simulink model "QuadrotorVertPlane_R2017b"  (R2020a)
settings: Solver=ode23s  StartTime=0.0  StopTime=20  RelTol=1e-3  EnableMultiTasking=on
values from neighbouring files (symbols this model uses):
  Acx = 4    [quadrotorparam.m]
  Acy = 4    [quadrotorparam.m]
  bt = 1    [quadrotorparam.m]
  ciLtheta = 0    [quadrotorparam.m]
  cipx = 0    [quadrotorparam.m]
  cipy = 0    [quadrotorparam.m]
  citheta = 0    [quadrotorparam.m]
  cix = 0    [quadrotorparam.m]
  ciy = 0    [quadrotorparam.m]
  g = 9.8    [quadrotorparam.m]
  J = 0.0112    [quadrotorparam.m]
  kt = 5    [quadrotorparam.m]
  kvt = 5    [quadrotorparam.m]
  kvx = .1    (= 0.1)    [quadrotorparam.m]
  kvy = 1    [quadrotorparam.m]
  kx = .5    (= 0.5)    [quadrotorparam.m]
  ky = .5    (= 0.5)    [quadrotorparam.m]
  l = 0.2    [quadrotorparam.m]
  lf = 0.2    [quadrotorparam.m]
  lr = 0.2    [quadrotorparam.m]
  m = 1    [quadrotorparam.m]
  SteptOff = 80    [quadrotorparam.m]
  SteptTc = 20    [quadrotorparam.m]
  Tcx = 30    [quadrotorparam.m]
  Tcy = 30    [quadrotorparam.m]
  txref = 1    [quadrotorparam.m]
  tyref = 1    [quadrotorparam.m]
  xref = 10    [quadrotorparam.m]
  yref = 10    [quadrotorparam.m]
settings Model: Creator=tristan  LastModifiedBy=cal
settings DataIOCC: SaveFormat=Array  SignalLoggingSaveFormat=ModelDataLogs  ReturnWorkspaceOutputs=off  OutputOption=SpecifiedOutputTimes  OutputTimes=[tStart:outputsample:tFinal]
settings OptimizationCC: ExpressionDepthLimit=2147483647  LifeSpan=inf
settings DebuggingCC: UnderspecifiedInitializationDetection=Classic  MergeDetectMultiDrivingBlocksExec=none  FcnCallInpInsideContextMsg=warning  StateNameClashWarn=warning  SFUnexpectedBacktrackingDiag=warning  SFNoUnconditionalDefaultTransitionDiag=warning  SFExecutionAtInitializationDiag=none  ArithmeticOperatorsInVariantConditions=warning
settings HardwareCC: ProdBitPerPointer=32  ProdBitPerSizeT=32  ProdBitPerPtrDiffT=32  ProdLargestAtomicFloat=None  ProdIntDivRoundTo=Undefined  ProdEndianess=Unspecified  ProdWordSize=32  ProdHWDeviceType=32-bit Generic
settings ModelReferenceCC: PropagateSignalLabelsOutOfModel=off
settings SFSimCC: SimUseLocalCustomCode=off  CustomCodeUndefinedFunction=UseInterfaceOnly
settings RTWCC: RTWUseLocalCustomCode=off
settings CodeAppCC: StateflowObjectComments=on
settings GRTTargetCC: TargetLangStandard=C89/C90 (ANSI)  CombineOutputUpdateFcns=off  GRTInterface=on
settings ConfigComp: CovMetricSettings=dw  CovHtmlReporting=on  CovSaveCumulativeToWorkspaceVar=on  CovSaveSingleToWorkspaceVar=on  CovExternalEMLEnable=off

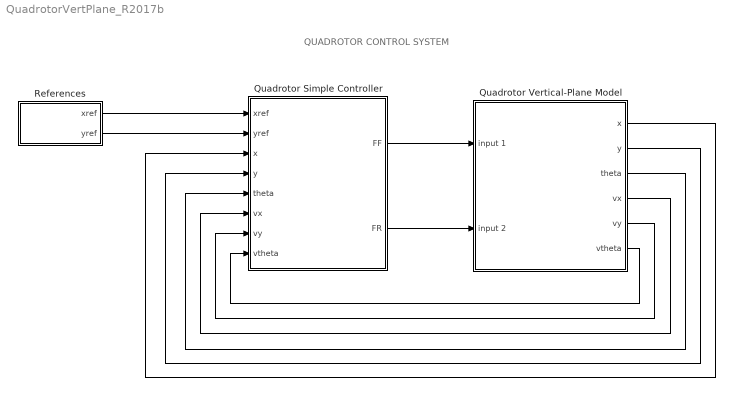
== system QuadrotorVertPlane_R2017b ==
  note: QUADROTOR CONTROL SYSTEM
  Quadrotor Simple Controller : Subsystem
  Quadrotor Vertical-Plane Model : Subsystem
  References : Subsystem
  wires:
  Quadrotor Vertical-Plane Model/3(theta) -> Quadrotor Simple Controller/5(theta)
  Quadrotor Vertical-Plane Model/2(y) -> Quadrotor Simple Controller/4(y)
  Quadrotor Vertical-Plane Model/1(x) -> Quadrotor Simple Controller/3(x)
  Quadrotor Simple Controller/1(FF) -> Quadrotor Vertical-Plane Model/1(input 1)
  Quadrotor Simple Controller/2(FR) -> Quadrotor Vertical-Plane Model/2(input 2)
  Quadrotor Vertical-Plane Model/5(vy) -> Quadrotor Simple Controller/7(vy)
  Quadrotor Vertical-Plane Model/4(vx) -> Quadrotor Simple Controller/6(vx)
  Quadrotor Vertical-Plane Model/6(vtheta) -> Quadrotor Simple Controller/8(vtheta)
  References/2(yref) -> Quadrotor Simple Controller/2(yref)
  References/1(xref) -> Quadrotor Simple Controller/1(xref)

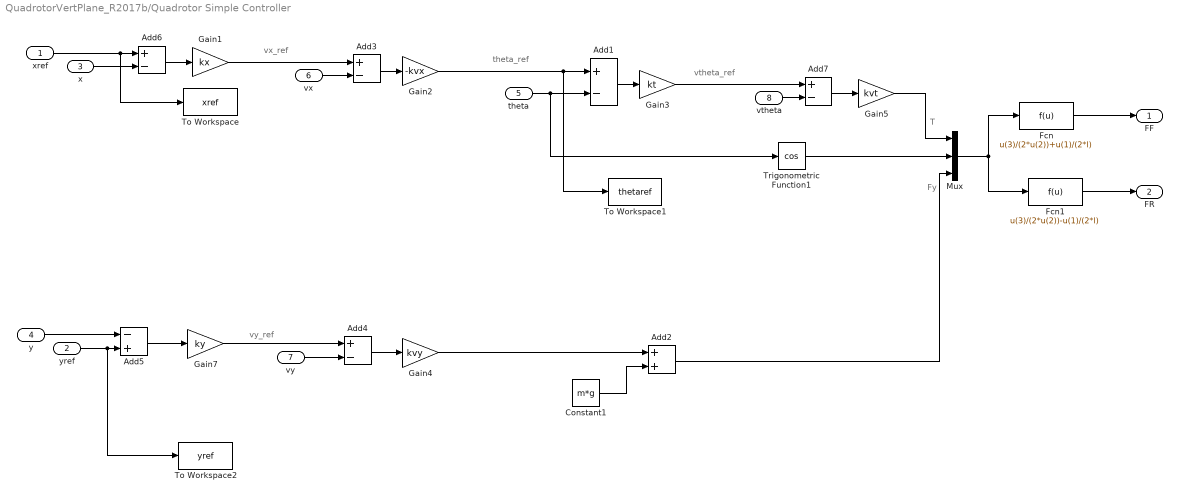
== system QuadrotorVertPlane_R2017b/Quadrotor Simple Controller ==
  note: T
  note: Fy
  note: vx_ref
  note: theta_ref
  note: vtheta_ref
  note: vy_ref
  xref : Inport
  yref : Inport  Port=2
  x : Inport  Port=3
  y : Inport  Port=4
  theta : Inport  Port=5
  vx : Inport  Port=6
  vy : Inport  Port=7
  vtheta : Inport  Port=8
  Add{1,3..4,6..7} (5 alike) : Sum  Inputs=+-
  Add2 : Sum
  Add5 : Sum  Inputs=-+
  Constant1 : Constant  Value=m*g
  Fcn : Fcn  Expr=u(3)/(2*u(2))+u(1)/(2*l)
  Fcn1 : Fcn  Expr=u(3)/(2*u(2))-u(1)/(2*l)
  Gain1 : Gain  Gain=kx
  Gain2 : Gain  Gain=-kvx
  Gain3 : Gain  Gain=kt
  Gain4 : Gain  Gain=kvy
  Gain5 : Gain  Gain=kvt
  Gain7 : Gain  Gain=ky
  Mux : Mux  Inputs=3
  To Workspace : ToWorkspace  VariableName=xref  SampleTime=-1
  To Workspace1 : ToWorkspace  VariableName=thetaref  SampleTime=-1
  To Workspace2 : ToWorkspace  VariableName=yref  SampleTime=-1
  Trigonometric Function1 : Trigonometry  Operator=cos
  FF : Outport  VectorParamsAs1DForOutWhenUnconnected=off
  FR : Outport  Port=2  VectorParamsAs1DForOutWhenUnconnected=off
  wires:
  x/1 -> Add6/2
  Add6/1 -> Gain1/1
  theta/1 -> Add1/2, Trigonometric Function1/1
  Add1/1 -> Gain3/1
  y/1 -> Add5/1
  Add5/1 -> Gain7/1
  Constant1/1 -> Add2/2
  Add2/1 -> Mux/3
  Trigonometric Function1/1 -> Mux/2
  Fcn/1 -> FF/1
  Fcn1/1 -> FR/1
  Mux/1 -> Fcn/1, Fcn1/1
  xref/1 -> To Workspace/1, Add6/1
  Gain2/1 -> To Workspace1/1, Add1/1
  yref/1 -> To Workspace2/1, Add5/2
  vx/1 -> Add3/2
  Add3/1 -> Gain2/1
  vy/1 -> Add4/2
  Add4/1 -> Gain4/1
  Gain7/1 -> Add4/1
  Gain4/1 -> Add2/1
  vtheta/1 -> Add7/2
  Add7/1 -> Gain5/1
  Gain3/1 -> Add7/1
  Gain1/1 -> Add3/1
  Gain5/1 -> Mux/1

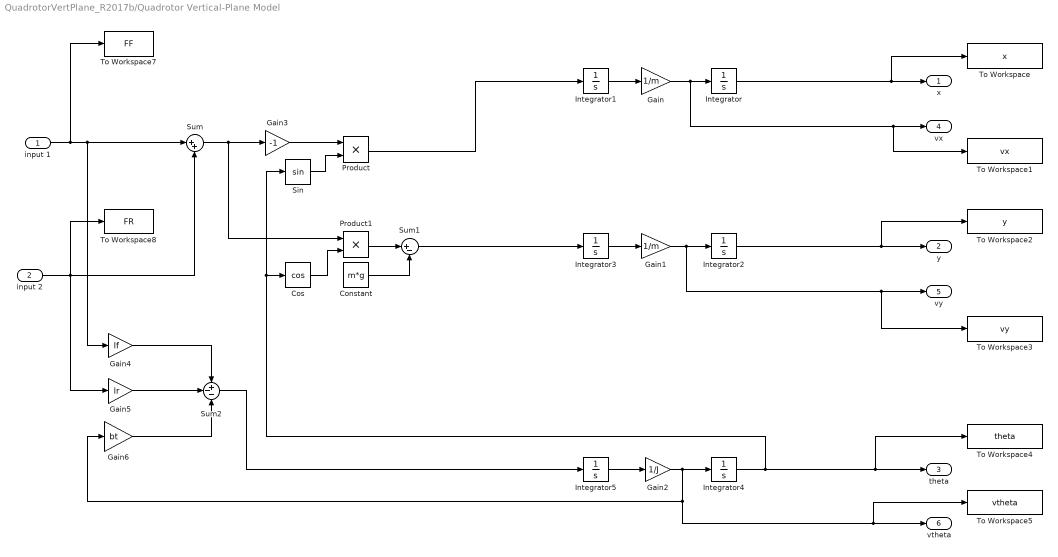
== system QuadrotorVertPlane_R2017b/Quadrotor Vertical-Plane Model ==
  input 1 : Inport
  input 2 : Inport  Port=2
  Constant : Constant  Value=m*g
  Cos : Trigonometry  Operator=cos
  Gain : Gain  Gain=1/m
  Gain1 : Gain  Gain=1/m
  Gain2 : Gain  Gain=1/J
  Gain3 : Gain  Gain=-1
  Gain4 : Gain  Gain=lf
  Gain5 : Gain  Gain=lr
  Gain6 : Gain  Gain=bt
  Integrator : Integrator  InitialCondition=cix
  Integrator1 : Integrator  InitialCondition=cipx
  Integrator2 : Integrator  InitialCondition=ciy
  Integrator3 : Integrator  InitialCondition=cipy
  Integrator4 : Integrator  InitialCondition=citheta
  Integrator5 : Integrator  InitialCondition=ciLtheta
  Product : Product
  Product1 : Product
  Sin : Trigonometry
  Sum : Sum  Inputs=|++
  Sum1 : Sum  Inputs=|+-
  Sum2 : Sum  Inputs=+--
  To Workspace : ToWorkspace  VariableName=x  SampleTime=-1
  To Workspace1 : ToWorkspace  VariableName=vx  SampleTime=-1
  To Workspace2 : ToWorkspace  VariableName=y  SampleTime=-1
  To Workspace3 : ToWorkspace  VariableName=vy  SampleTime=-1
  To Workspace4 : ToWorkspace  VariableName=theta  SampleTime=-1
  To Workspace5 : ToWorkspace  VariableName=vtheta  SampleTime=-1
  To Workspace7 : ToWorkspace  VariableName=FF  SampleTime=-1
  To Workspace8 : ToWorkspace  VariableName=FR  SampleTime=-1
  x : Outport  VectorParamsAs1DForOutWhenUnconnected=off
  y : Outport  Port=2  VectorParamsAs1DForOutWhenUnconnected=off
  theta : Outport  Port=3  VectorParamsAs1DForOutWhenUnconnected=off
  vx : Outport  Port=4  VectorParamsAs1DForOutWhenUnconnected=off
  vy : Outport  Port=5  VectorParamsAs1DForOutWhenUnconnected=off
  vtheta : Outport  Port=6  VectorParamsAs1DForOutWhenUnconnected=off
  wires:
  Integrator1/1 -> Gain/1
  Gain/1 -> Integrator/1, To Workspace1/1, vx/1
  Integrator3/1 -> Gain1/1
  Gain1/1 -> Integrator2/1, To Workspace3/1, vy/1
  Integrator5/1 -> Gain2/1
  Gain2/1 -> Integrator4/1, To Workspace5/1, vtheta/1, Gain6/1
  Integrator4/1 -> Sin/1, Cos/1, To Workspace4/1, theta/1
  Integrator/1 -> To Workspace/1, x/1
  Integrator2/1 -> To Workspace2/1, y/1
  input 1/1 -> Gain4/1, Sum/1, To Workspace7/1
  input 2/1 -> Gain5/1, Sum/2, To Workspace8/1
  Sum/1 -> Product1/1, Gain3/1
  Sin/1 -> Product/2
  Gain3/1 -> Product/1
  Cos/1 -> Product1/2
  Product1/1 -> Sum1/1
  Constant/1 -> Sum1/2
  Product/1 -> Integrator1/1
  Sum1/1 -> Integrator3/1
  Gain6/1 -> Sum2/3
  Gain5/1 -> Sum2/2
  Gain4/1 -> Sum2/1
  Sum2/1 -> Integrator5/1

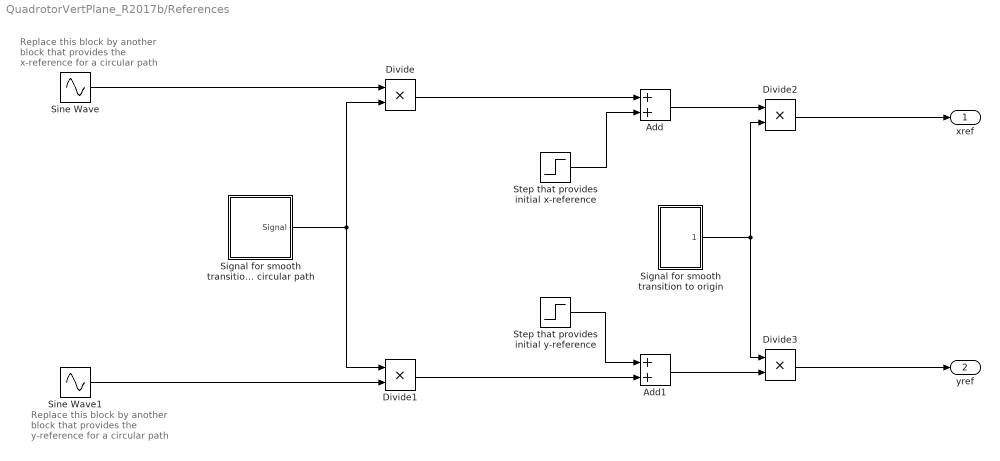
== system QuadrotorVertPlane_R2017b/References ==
  note: Replace this block by another block that provides the x-reference for a circular path
  note: Replace this block by another block that provides the y-reference for a circular path
  Add : Sum
  Add1 : Sum
  Divide{,1..3} (4 alike) : Product  Inputs=**
  Signal for smooth transition to circular path : Subsystem
  Signal for smooth transition to origin : Subsystem
  Sine Wave : Sin  Amplitude=Acx  Frequency=2 * pi / Tcx  SampleTime=0
  Sine Wave1 : Sin  Amplitude=Acy  Frequency=2 * pi / Tcy  Phase=pi / 2  SampleTime=0
  "Step that provides initial x-reference " : Step  Time=txref  After=xref  SampleTime=0
  "Step that provides initial y-reference " : Step  Time=tyref  After=yref  SampleTime=0
  xref : Outport  VectorParamsAs1DForOutWhenUnconnected=off
  yref : Outport  Port=2  VectorParamsAs1DForOutWhenUnconnected=off
  wires:
  "Step that provides initial x-reference "/1 -> Add/2
  "Step that provides initial y-reference "/1 -> Add1/1
  Divide/1 -> Add/1
  Divide1/1 -> Add1/2
  Add/1 -> Divide2/1
  Divide3/1 -> yref/1
  Add1/1 -> Divide3/2
  Divide2/1 -> xref/1
  Signal for smooth transition to circular path/1(Signal) -> Divide/2, Divide1/1
  Signal for smooth transition to origin/1(Signal) -> Divide2/2, Divide3/1
  Sine Wave/1 -> Divide/1
  Sine Wave1/1 -> Divide1/2

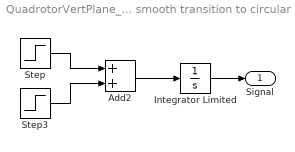
== system QuadrotorVertPlane_R2017b/References/Signal for smooth transition to circular path ==
  Add2 : Sum
  Integrator Limited : Integrator  LimitOutput=on  UpperSaturationLimit=1  LowerSaturationLimit=0
  Step : Step  Time=SteptTc  After=0.1  SampleTime=0
  Step3 : Step  Time=SteptOff  After=.8  SampleTime=0
  Signal : Outport  VectorParamsAs1DForOutWhenUnconnected=off
  wires:
  Integrator Limited/1 -> Signal/1
  Add2/1 -> Integrator Limited/1
  Step/1 -> Add2/1
  Step3/1 -> Add2/2

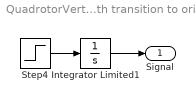
== system QuadrotorVertPlane_R2017b/References/Signal for smooth transition to origin ==
  Integrator Limited1 : Integrator  InitialCondition=1  LimitOutput=on  UpperSaturationLimit=1  LowerSaturationLimit=0
  Step4 : Step  Time=SteptOff  After=-0.05  SampleTime=0
  Signal : Outport  VectorParamsAs1DForOutWhenUnconnected=off
  wires:
  Integrator Limited1/1 -> Signal/1
  Step4/1 -> Integrator Limited1/1
